simulink model "gm_test_prediction_without_delays"  (R2022a)
settings: Solver=FixedStepDiscrete  StartTime=0.0  StopTime=10.0  RelTol=1e-3
undefined symbols (not defined in the file or in its folder): f_c, L_d, L_q, L_x, L_y, p, psi_pm, R_ph
libraries: hdlmdlgenlib x2
(part 1 of 9)
settings Model: Creator=Andre Merx  LastModifiedBy=Andre Merx
settings SolverCC: AlgebraicLoopSolver=TrustRegion
settings DataIOCC: LimitDataPoints=on  SaveOutput=off  SaveTime=off
settings OptimizationCC: BlockReduction=off  ConditionallyExecuteInputs=off  DefaultParameterBehavior=Inlined  LifeSpan=inf
settings DebuggingCC: AlgebraicLoopMsg=error  InheritedTsInSrcMsg=none  SingleTaskRateTransMsg=error  UnconnectedInputMsg=warning  UnconnectedOutputMsg=warning  UnconnectedLineMsg=warning  AllowSymbolicDim=off  StrictBusMsg=ErrorOnBusTreatedAsVector  SFUnexpectedBacktrackingDiag=warning  SFNoUnconditionalDefaultTransitionDiag=warning  SFExecutionAtInitializationDiag=none  SFMachineParentedDataDiag=warning  ArithmeticOperatorsInVariantConditions=warning
settings HardwareCC: ProdBitPerPointer=32  ProdBitPerSizeT=32  ProdBitPerPtrDiffT=32  ProdLargestAtomicFloat=None  ProdIntDivRoundTo=Undefined  ProdEndianess=Unspecified  ProdWordSize=32  ProdHWDeviceType=ASIC/FPGA->ASIC/FPGA  ProdEqTarget=off
settings SFSimCC: SimUseLocalCustomCode=off  CustomCodeUndefinedFunction=UseInterfaceOnly
settings RTWCC: RTWUseLocalCustomCode=off
settings CodeAppCC: StateflowObjectComments=on
settings GRTTargetCC: TargetLangStandard=C89/C90 (ANSI)
settings ConfigComp: CovScope=ReferencedModels  CovMetricSettings=dw  CovSaveCumulativeToWorkspaceVar=on  CovSaveSingleToWorkspaceVar=on  CovExternalEMLEnable=off  CovSFcnEnable=off

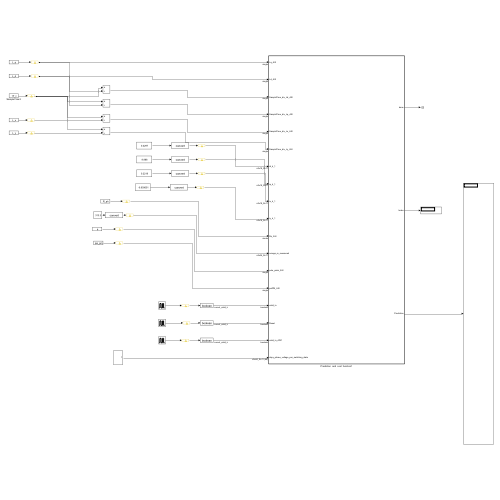
[thumbnail: Simulink's stored preview of the top-level diagram]
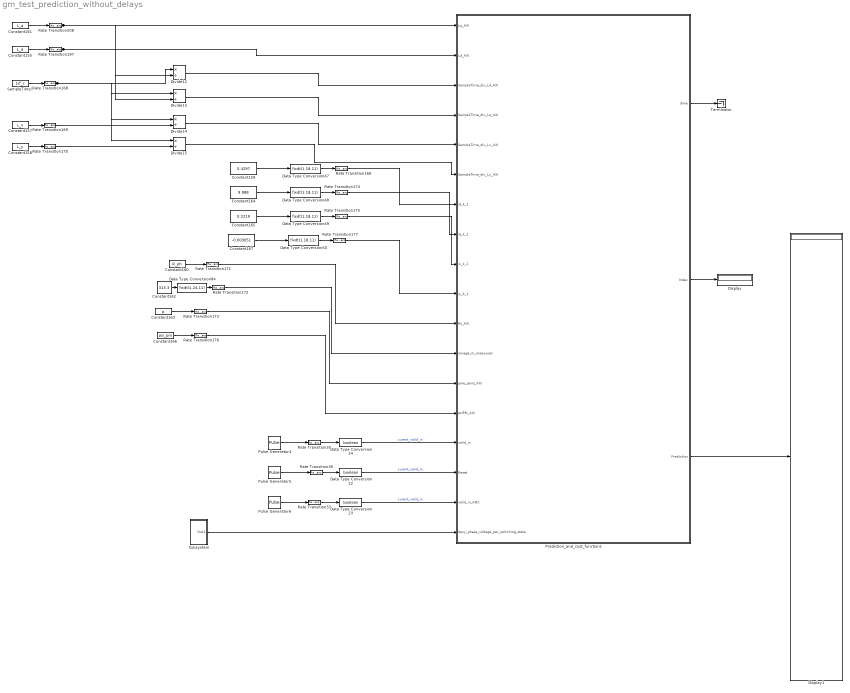
== system gm_test_prediction_without_delays ==
  Constant155 : Constant  Value=L_d  OutDataTypeStr=single  SampleTime=-1
  Constant157 : Constant  Value=L_x  OutDataTypeStr=single  SampleTime=-1
  Constant158 : Constant  Value=L_y  OutDataTypeStr=single  SampleTime=-1
  Constant159 : Constant  Value=0.4297
  Constant160 : Constant  Value=R_ph  OutDataTypeStr=single  SampleTime=-1
  Constant161 : Constant  Value=L_q  OutDataTypeStr=single  SampleTime=-1
  Constant162 : Constant  Value=313.3
  Constant163 : Constant  Value=p  OutDataTypeStr=single  SampleTime=-1
  Constant164 : Constant  Value=9.988
  Constant165 : Constant  Value=0.2219
  Constant166 : Constant  Value=psi_pm  OutDataTypeStr=single  SampleTime=-1
  Constant167 : Constant  Value=-0.003051
  Data Type Conversion22 : DataTypeConversion  OutDataTypeStr=boolean  SaturateOnIntegerOverflow=off  RndMeth=Floor
  Data Type Conversion23 : DataTypeConversion  OutDataTypeStr=boolean  SaturateOnIntegerOverflow=off  RndMeth=Floor
  Data Type Conversion24 : DataTypeConversion  OutDataTypeStr=boolean  SaturateOnIntegerOverflow=off  RndMeth=Floor
  Data Type Conversion{47..50} (4 alike) : DataTypeConversion  OutDataTypeStr=fixdt(1,18,11)  SaturateOnIntegerOverflow=off  RndMeth=Floor
  Data Type Conversion84 : DataTypeConversion  OutDataTypeStr=fixdt(1,24,11)  SaturateOnIntegerOverflow=off  RndMeth=Floor
  Display : Display
  Display1 : Display
  Divide{12..15} (4 alike) : Product  Inputs=*/  RndMeth=Zero  SaturateOnIntegerOverflow=on
  Prediction_and_cost_function1 : Subsystem  TreatAsAtomicUnit=on
  Pulse Generator4 : DiscretePulseGenerator  PulseType=Time based  Period=1/f_c
  Pulse Generator5 : DiscretePulseGenerator  PulseType=Time based  Period=1/f_c
  Pulse Generator6 : DiscretePulseGenerator  PulseType=Time based  Period=1/f_c
  Rate Transition{35..37,166,168..177,197,208} (16 alike) : RateTransition  OutPortSampleTime=Rt
  SampleTime3 : Constant  Value=1/f_c  OutDataTypeStr=single  SampleTime=-1
  Subsystem : Subsystem
  Terminator : Terminator
  wires:
  Prediction_and_cost_function1/3(Prediction) -> Display1/1
  Prediction_and_cost_function1/2(Index) -> Display/1
  Prediction_and_cost_function1/1(done) -> Terminator/1
  Rate Transition35/1 -> Data Type Conversion24/1
  Data Type Conversion22/1 -> Prediction_and_cost_function1/16(Reset)  "curent_valid_in"
  Rate Transition36/1 -> Data Type Conversion22/1
  Data Type Conversion24/1 -> Prediction_and_cost_function1/15(valid_in)  "curent_valid_in"
  Data Type Conversion23/1 -> Prediction_and_cost_function1/17(valid_in_ADC)  "curent_valid_in"
  Rate Transition37/1 -> Data Type Conversion23/1
  Pulse Generator4/1 -> Rate Transition35/1
  Pulse Generator5/1 -> Rate Transition36/1
  Pulse Generator6/1 -> Rate Transition37/1
  Rate Transition166/1 -> Prediction_and_cost_function1/7(id_k_1)
  Constant161/1 -> Rate Transition208/1
  Divide12/1 -> Prediction_and_cost_function1/3(SampleTime_div_Ld_AXI)
  Data Type Conversion49/1 -> Rate Transition175/1
  Rate Transition173/1 -> Prediction_and_cost_function1/13(pole_pairs_AXI)
  Constant158/1 -> Rate Transition170/1
  Rate Transition170/1 -> Divide15/2
  Constant157/1 -> Rate Transition169/1
  Constant159/1 -> Data Type Conversion47/1
  Rate Transition171/1 -> Prediction_and_cost_function1/11(Rs_AXI)
  Data Type Conversion50/1 -> Rate Transition177/1
  Rate Transition169/1 -> Divide14/2
  Divide14/1 -> Prediction_and_cost_function1/5(SampleTime_div_Lx_AXI)
  Data Type Conversion47/1 -> Rate Transition166/1
  SampleTime3/1 -> Rate Transition168/1
  Rate Transition172/1 -> Prediction_and_cost_function1/12(omega_m_measured)
  Constant164/1 -> Data Type Conversion48/1
  Rate Transition197/1 -> Prediction_and_cost_function1/2(Ld_AXI), Divide12/2
  Rate Transition208/1 -> Prediction_and_cost_function1/1(Lq_AXI), Divide13/2
  Rate Transition168/1 -> Divide12/1, Divide14/1, Divide15/1, Divide13/1
  Divide13/1 -> Prediction_and_cost_function1/4(SampleTime_div_Lq_AXI)
  Rate Transition177/1 -> Prediction_and_cost_function1/10(iy_k_1)
  Constant162/1 -> Data Type Conversion84/1
  Constant155/1 -> Rate Transition197/1
  Constant163/1 -> Rate Transition173/1
  Rate Transition175/1 -> Prediction_and_cost_function1/9(ix_k_1)
  Rate Transition176/1 -> Prediction_and_cost_function1/14(psiPM_AXI)
  Data Type Conversion84/1 -> Rate Transition172/1
  Constant160/1 -> Rate Transition171/1
  Constant166/1 -> Rate Transition176/1
  Constant165/1 -> Data Type Conversion49/1
  Constant167/1 -> Data Type Conversion50/1
  Rate Transition174/1 -> Prediction_and_cost_function1/8(iq_k_1)
  Subsystem/1(Out1) -> Prediction_and_cost_function1/18(dqxy_phase_voltage_per_switching_state)
  Data Type Conversion48/1 -> Rate Transition174/1
  Divide15/1 -> Prediction_and_cost_function1/6(SampleTime_div_Ly_AXI)
